simulink model "ACC_adptv_MPC_augment_constr_accel_inpt_ateteemp"  (R2024a)
settings: Solver=FixedStepAuto  StartTime=0  StopTime=100  FixedStep=.05  RelTol=1e-3
undefined symbols (not defined in the file or in its folder): act_t_delay, aero_const, ctrl_batch, Defined, delta_U_max, delta_U_min, driver_set_spd, Ego, Lane, m, matlabshared, N, Qbar, Rbar, simStepSize, state_batch, U_max, U_min, User, Y_max, Y_min
libraries: roadrunnerscenario x4, drivingscenarioandsensors x1, autolibshared x1
settings Model: PacingRate=10  Creator=darkh  LastModifiedBy=darkh
settings DataIOCC: ReturnWorkspaceOutputsName=sltest_internal_rrSimulationOutputVariable
settings DebuggingCC: AlgebraicLoopMsg=none
settings RTWCC: GPUComputeCapability=3.5
settings ConfigComp: CovSaveName=sltest_covdata  CovMetricSettings=dcmwe  CovEnableCumulative=off  CovSaveSingleToWorkspaceVar=on  CovSaveOutputData=off

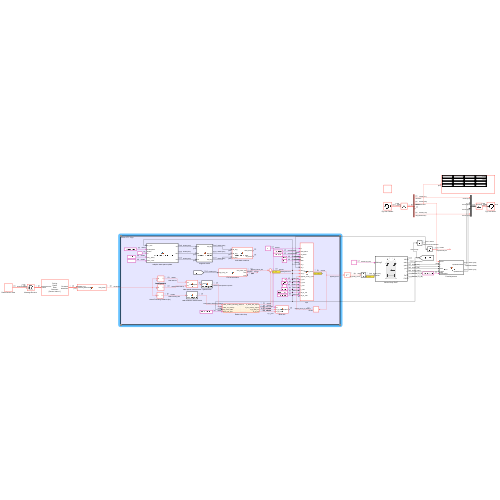
[thumbnail: Simulink's stored preview of the top-level diagram]
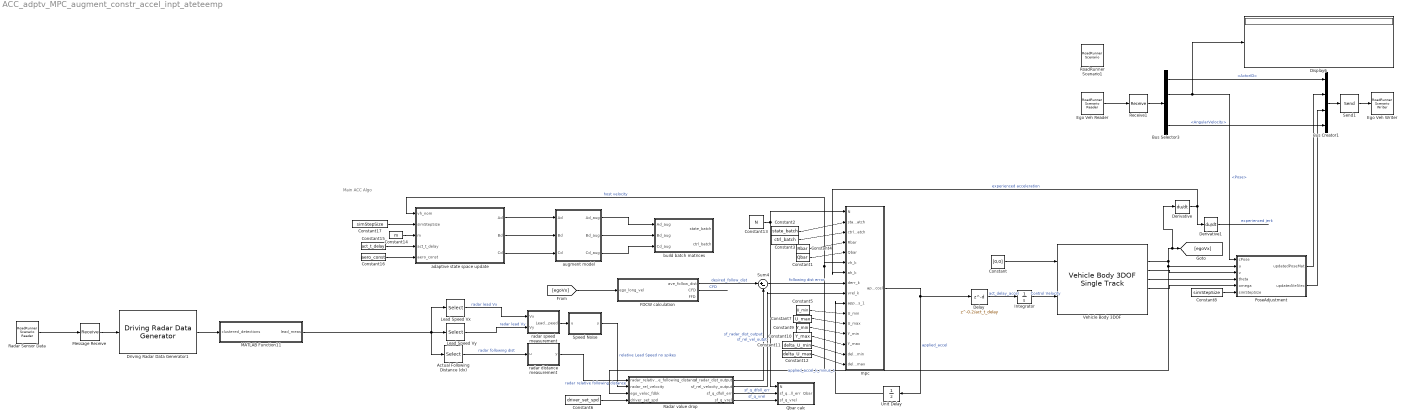
== system ACC_adptv_MPC_augment_constr_accel_inpt_ateteemp ==
  note: Main ACC Algo
  Actual Following Distance (dx) : Selector  InputPortWidth=6  IndexOptions=Index vector (dialog)  Indices=[1]  OutputSizes=1
  Bus Creator1 : BusCreator  Inputs=4  OutDataTypeStr=Bus: BusActorRuntime  NonVirtualBus=on
      settings: InheritFromInputs=off
  Bus Selector3 : BusSelector  OutputSignals=ActorID,Pose,Velocity,AngularVelocity
  Constant : Constant  Value=[0,0]
  Constant1 : Constant  Value=Qbar
  Constant10 : Constant  Value=Y_max
  Constant11 : Constant  Value=delta_U_min
  Constant12 : Constant  Value=delta_U_max
  Constant13 : Constant  Value=N
  Constant14 : Constant  Value=m
  Constant15 : Constant  Value=act_t_delay
  Constant16 : Constant  Value=aero_const
  Constant17 : Constant  Value=simStepSize
  Constant2 : Constant  Value=state_batch
  Constant3 : Constant  Value=ctrl_batch
  Constant4 : Constant  Value=Rbar
  Constant5 : Constant  Value=U_min
  Constant6 : Constant  Value=driver_set_spd
  Constant7 : Constant  Value=U_max
  Constant8 : Constant  Value=simStepSize
  Constant9 : Constant  Value=Y_min
  Delay : Delay  DelayLength=0.2/act_t_delay
  Derivative : Derivative
  Derivative1 : Derivative
  Display6 : Display
  Driving Radar Data Generator1 : drivingscenarioandsensors/Driving Radar Data Generator  SensorIndex=1  UpdateRate=20  MountingLocation=[ 3.4, 0, 0.2 ]  MountingAngles=[0 0 0]  HasElevation=off  HasRangeRate=on  HasNoise=on  HasFalseAlarms=on  HasOcclusion=on  MaxNumReportsSource=Property  MaxNumReports=50  TargetReportFormat=Clustered detections  DetectionCoordinates=Body  TrackCoordinates=Body  BusNameSource=Auto  BusName=BusDrivingRadarDataGenerator  AzimuthResolution=4  ElevationResolution=5  RangeResolution=2.5  RangeRateResolution=0.5  AzimuthBiasFraction=0.1  ElevationBiasFraction=0.1  RangeBiasFraction=0.05  RangeRateBiasFraction=0.05  FieldOfView=[ 20, 5 ]  RangeLimits=[ 0, 150 ]  RangeRateLimits=[ -100, 100 ]  DetectionProbability=0.9  FalseAlarmRate=1e-06  ReferenceRange=100  ReferenceRCS=0  CenterFrequency=77e9  FilterInitializationFcn=initcvekf  ConfirmationThreshold=[2 3]  DeletionThreshold=[5 5]  InitialSeedSource=Repeatable  InitialSeed=0  UsedSeed=matlabshared.tracking.internal.SimulinkUtilities.seedManager(gcb)  ProfilesSource=From Scenario Reader block  ProfilesParameters=driving.internal.ActorProfilesRadarParameters  ProfilesExpression=struct('ClassID',0,'Length',4.7,'Width',1.8,'Height',1.4,'OriginOffset',[-1.35 0 0],'RCSPattern',[10 10;10 10],'RCSAzimuthAngles',[-180 180],'RCSElevationAngles',[-90 90])
  Ego Veh Reader : roadrunnerscenario/RoadRunner Scenario Reader  TopicCategory=Actor  ActorCategory=All Types  ActionType=Path Following  EventType=User-Defined  TopicType=Actor Pose  VehicleType=Vehicle Specifications  UserDefinedAction=Action1  UserDefinedEvent=Event1  Filter=Self  SensorTopic=Target Poses  LaneBoundaryOutputTopic=Ego-Lane  SensorID=1  SampleTime=simStepSize
  Ego Veh Writer : roadrunnerscenario/RoadRunner Scenario Writer  TopicCategory=Actor  ActorCategory=All Types  EventType=Action Complete  UserDefinedEvent=Event1  VehicleType=Vehicle Pose  TopicType=Actor Pose
  FDCW calculation : MATLAB Function  TreatAsAtomicUnit=on
  Integrator : Integrator
  Lead Speed Vx : Selector  InputPortWidth=6  IndexOptions=Index vector (dialog)  Indices=4  OutputSizes=1
  Lead Speed Vy : Selector  InputPortWidth=6  IndexOptions=Index vector (dialog)  Indices=5  OutputSizes=1
  MATLAB Function11 : MATLAB Function  TreatAsAtomicUnit=on
  Message Receive : Receive  InputPortMessageModes=m  UseInternalQueue=off
  PoseAdjustment : MATLAB Function  TreatAsAtomicUnit=on
  Qbar calc : MATLAB Function  TreatAsAtomicUnit=on  SystemSampleTime=simStepSize
  Radar Sensor Data : roadrunnerscenario/RoadRunner Scenario Reader  TopicCategory=Sensor  ActorCategory=All Types  ActionType=Path Following  EventType=User-Defined  TopicType=Actor Specifications  VehicleType=Vehicle Specifications  UserDefinedAction=Action1  UserDefinedEvent=Event1  Filter=Self  SensorTopic=Target Poses  LaneBoundaryOutputTopic=Ego-Lane  SensorID=1  SampleTime=simStepSize
  Radar value drop : Stateflow chart  TreatAsAtomicUnit=on
  Receive1 : Receive  InputPortMessageModes=m  UseInternalQueue=off  QueueOverwriting=on  QueueLength=1  QueueType=LIFO
  RoadRunner Scenario1 : roadrunnerscenario/RoadRunner Scenario  UserDefinedActions={}  UserDefinedEvents={}
  Send1 : Send  OutputPortMessageModes=m
  Speed Noise : MATLAB Function  TreatAsAtomicUnit=on
  Sum4 : Sum  Inputs=|+-
  Unit Delay : UnitDelay  SampleTime=-1  HasFrameUpgradeWarning=on
  "Vehicle Body 3DOF " : autolibshared/Vehicle Body 3DOF Single Track  trackMode=Dual  inputMode=External longitudinal velocity  frontSteerMode=on  rearSteerMode=off  windMode=off  muMode=off  extFMode=off  extMMode=off  htchFMode=off  htchMMode=off  extXo=off  extpsio=off  extxdoto=off  extro=off  extYo=off  extTamb=off  extydoto=off  aMode=2  NF=2  NR=2  m=m  a=1.5569  b=1.5371  h=0.18903  dh=1  hh=0.2  X_o=0  xdot_o=0  CalphaMode=off  sigmaMode=on  d=0  hl=0  w=[1.4,1.4]  Cy_f=40000  Cy_r=40000  sigma_f=.1  sigma_r=.1  alpha_f_brk=[-.1 .1]  Cy_f_data=[-9e3 9e3]  alpha_r_brk=[-.1 .1]  Cy_r_data=[-9e3 9e3]  Y_o=0  ydot_o=0  Izz=2066  psi_o=0  r_o=0  Af=2.73  Cd=.30356  Cl=.1  Cpm=.1  beta_w=[0 0.01:0.01:0.3]  Cs=[0 0.01:0.01:0.3]  Cym=[0 1e-6:0.01:0.3]  Pabs=101325  Tair=273  g=9.81  mu=1  xdot_tol=.01  Fznom=5000  Fxtire_sat=7e4  Fytire_sat=7e4  longOff=0  latOff=0  vertOff=0  wrapAng=off
  adaptive state space update : MATLAB Function  TreatAsAtomicUnit=on
  augment model : MATLAB Function  TreatAsAtomicUnit=on
  build batch matrices : MATLAB Function  TreatAsAtomicUnit=on  SystemSampleTime=simStepSize
  mpc : MATLAB Function  TreatAsAtomicUnit=on  SystemSampleTime=simStepSize
  radar distance measurement : MATLAB Function  TreatAsAtomicUnit=on
  radar speed measurement : MATLAB Function  TreatAsAtomicUnit=on
  wires:
  Bus Selector3/4 -> Bus Creator1/4  "<AngularVelocity>"
  Bus Creator1/1 -> Send1/1
  Bus Selector3/1 -> Bus Creator1/1  "<ActorID>"
  Receive1/1 -> Bus Selector3/1
  Send1/1 -> Ego Veh Writer/1
  Ego Veh Reader/1 -> Receive1/1
  Bus Selector3/2 -> Display6/1, PoseAdjustment/1(cPose)  "<Pose>"
  PoseAdjustment/1(updatedPoseMat) -> Bus Creator1/2
  "Vehicle Body 3DOF "/2 -> PoseAdjustment/2(u), Radar value drop/3(ego_veloc_fdbk), adaptive state space update/1(vh_nom), mpc/6(vh_k), Derivative/1, [egoVx]  "host velocity"
  Radar Sensor Data/1 -> Message Receive/1
  Message Receive/1 -> Driving Radar Data Generator1/1
  Driving Radar Data Generator1/1 -> MATLAB Function11/1(clustered_detections)
  PoseAdjustment/2(updatedVelVec) -> Bus Creator1/3
  Integrator/1 -> "Vehicle Body 3DOF "/2  "Control Velocity"
  Constant/1 -> "Vehicle Body 3DOF "/1
  Sum4/1 -> mpc/8(derr_k)  "following dist error"
  Speed Noise/1(y) -> Radar value drop/2(radar_rel_velocity)  "relative Lead Speed no spikes"
  Lead Speed Vx/1 -> radar speed measurement/1(Vx)  "radar lead Vx"
  [egoVx] -> FDCW calculation/1(ego_long_vel)
  FDCW calculation/1(ave_follow_dist) -> Sum4/1  "desired_follow_dist"
  MATLAB Function11/1(lead_meas) -> Actual Following Distance (dx)/1, Lead Speed Vx/1, Lead Speed Vy/1
  radar distance measurement/1(y) -> Radar value drop/1(radar_relative_following_distance)  "radar relative following distance"
  Lead Speed Vy/1 -> radar speed measurement/2(Vy)  "radar lead Vy"
  radar speed measurement/1(LeadSpeed) -> Speed Noise/1(u)
  FDCW calculation/2(CFD) -> ?  "CFD"
  Actual Following Distance (dx)/1 -> radar distance measurement/1(u)  "radar following dist"
  Derivative/1 -> mpc/7(ah_k), Derivative1/1  "experienced acceleration"
  Derivative1/1 -> ?  "experienced jerk"
  Constant4/1 -> mpc/4(Rbar)
  Radar value drop/1(sf_radar_dist_output) -> Sum4/2  "sf_radar_dist_output"
  Constant6/1 -> Radar value drop/4(driver_set_spd)
  Radar value drop/2(sf_rel_velocity_output) -> mpc/9(vrel_k)  "sf_rel_vel_outpt"
  Radar value drop/3(sf_q_dfoll_err) -> Qbar calc/2(sf_q_dfoll_err)  "sf_q_dfoll_err"
  Radar value drop/4(sf_q_vrel) -> Qbar calc/3(sf_q_vrel)  "sf_q_vrel"
  Unit Delay/1 -> mpc/10(applied_accel_k_minus_1)  "applied_accel_k_minus_1"
  Constant5/1 -> mpc/11(U_min)
  Constant7/1 -> mpc/12(U_max)
  Constant8/1 -> PoseAdjustment/6(simStepSize)
  Constant9/1 -> mpc/13(Y_min)
  Constant10/1 -> mpc/14(Y_max)
  Constant11/1 -> mpc/15(del_U_min)
  Constant12/1 -> mpc/16(del_U_max)
  "Vehicle Body 3DOF "/4 -> PoseAdjustment/4(theta)
  Constant1/1 -> mpc/5(Qbar)
  "Vehicle Body 3DOF "/5 -> PoseAdjustment/5(omega)
  "Vehicle Body 3DOF "/3 -> PoseAdjustment/3(v)
  mpc/1(applied_accel) -> Unit Delay/1, Delay/1  "applied_accel"
  Constant14/1 -> adaptive state space update/3(m)
  Constant15/1 -> adaptive state space update/4(act_t_delay)
  Constant16/1 -> adaptive state space update/5(aero_const)
  Constant17/1 -> adaptive state space update/2(simStepSize)
  augment model/3(Cd_aug) -> build batch matrices/3(Cd_aug)
  augment model/2(Bd_aug) -> build batch matrices/2(Bd_aug)
  augment model/1(Ad_aug) -> build batch matrices/1(Ad_aug)
  Constant13/1 -> mpc/1(N), Qbar calc/1(N)
  adaptive state space update/1(Ad) -> augment model/1(Ad)
  adaptive state space update/2(Bd) -> augment model/2(Bd)
  adaptive state space update/3(Cd) -> augment model/3(Cd)
  Constant2/1 -> mpc/2(state_batch)
  Constant3/1 -> mpc/3(ctrl_batch)
  Delay/1 -> Integrator/1  "act_delay_accel"

== matlab function ACC_adptv_MPC_augment_constr_accel_inpt_ateteemp/build batch matrices ==
  data: state_batch output; Ad_aug input; Bd_aug input; Cd_aug input; ctrl_batch output
function [state_batch,ctrl_batch] = batch_matrix_build(Ad_aug,Bd_aug,Cd_aug)
[ny1,ny2] = size(Cd_aug);
[~,nu] = size(Bd_aug);

N=20;

% Building batch matrices for MPC prediction of output states
% batch matrix for state vector
state_batch = zeros(N*ny1, ny2);
for i = 1:N
    state_batch((i-1)*ny1+1 : i*ny1, :) = Cd_aug*(Ad_aug^i);
end

% Batch matrix for control vector
ctrl_batch = zeros(N*ny1, N*nu); % pre-allocate, fixed size

Apow = eye(size(Ad_aug)); % A^0
for i = 1:N
    % first column block for row i
    ctrl_batch((i-1)*ny1+(1:ny1), 1:nu) = Cd_aug*Apow*Bd_aug;
    % copy to the right for j = 2…i
    col = nu; % offset for next column
    Apow_j = Apow;
    for j = 2:i
        Apow_j = Apow_j / Ad_aug; % A^(i-j) (cheaper than repeated power)
        ctrl_batch((i-1)*ny1+(1:ny1), (j-1)*nu+(1:nu)) = Cd_aug*Apow_j*Bd_aug;
        col = col + nu;
    end
    Apow = Apow*Ad_aug; % advance A^i
end

== matlab function ACC_adptv_MPC_augment_constr_accel_inpt_ateteemp/PoseAdjustment ==
  data: cPose input; u input; updatedPoseMat output; v input; theta input; omega input; updatedVelVec output; simStepSize input
function [updatedPoseMat, updatedVelVec] = RRPoseAdjustment(cPose, u, v, theta, omega, simStepSize)
    thetad = theta + omega*simStepSize;
    xd = (u*cos(theta) - v*sin(theta))*simStepSize;
    yd = (u*sin(theta) + v*cos(theta))*simStepSize;
    pose_mat = [cos(-thetad) -sin(-thetad) 0 (yd+cPose(1,4)); sin(-thetad) cos(-thetad) 0 (xd+cPose(2,4)); 0 0 1 0; 0 0 0 1];
    updatedPoseMat = pose_mat;
    updatedVelVec = [u*sin(theta) + v*cos(theta), u*cos(theta) - v*sin(theta), 0];
    return;
end

== matlab function ACC_adptv_MPC_augment_constr_accel_inpt_ateteemp/radar distance measurement ==
  data: u input; y output
function y = removeSpikes(u)

    persistent buffer;
    persistent bufferIndex;
    threshold = 2;
    % windowSize = 15;
    windowSize = 5;
    
    if isempty(buffer)
        buffer = zeros(1, windowSize);
        bufferIndex = 1;
    end
    
    % Update buffer with new value
    buffer(bufferIndex) = u;
    bufferIndex = mod(bufferIndex, windowSize) + 1;
    
    % Calculate the median of the buffer
    medVal = median(buffer);
    
    % Detect and remove spikes
    if abs(u - medVal) > threshold
        y = medVal; % Replace spike with the median value
    else
        y = u; % Keep the original value if it's not a spike
    end
end

== matlab function ACC_adptv_MPC_augment_constr_accel_inpt_ateteemp/radar speed measurement ==
  data: Vx input; LeadSpeed output; Vy input
function LeadSpeed = fcn(Vx, Vy)

if Vx == 0 && Vy == 0 
    Vx = 0.01;
    Vy = 0.01;
elseif Vy == 0
    Vy = 0.01;
elseif Vx == 0
    Vx = 0.01;
end

if Vx <= 0
    LeadSpeed = -sqrt(Vx^2 + Vy^2);
else
    LeadSpeed = sqrt(Vx^2 + Vy^2);
end

== matlab function ACC_adptv_MPC_augment_constr_accel_inpt_ateteemp/Speed Noise ==
  settings: updateMethod=DISCRETE
  data: u input; y output
function y = removeSpikes(u)
    % removeSpikes - Removes spikes from a scalar signal based on a threshold
    %
    % Inputs:
    %    u - The input signal (scalar)
    %    threshold - The threshold value to detect spikes
    %    windowSize - The size of the window for calculating the median
    %
    % Outputs:
    %    y - The filtered signal with spikes removed

    % Declare persistent variables to store past values
    persistent buffer;
    persistent bufferIndex;
    threshold = 2;
    % windowSize = 15;
    windowSize = 5;

    
    if isempty(buffer)
        buffer = zeros(1, windowSize);
        bufferIndex = 1;
    end
    
    % Update buffer with new value
    buffer(bufferIndex) = u;
    bufferIndex = mod(bufferIndex, windowSize) + 1;
    
    % Calculate the median of the buffer
    medVal = median(buffer);
    
    % Detect and remove spikes
    if abs(u - medVal) > threshold
        y = medVal; % Replace spike with the median value
    else
        y = u; % Keep the original value if it's not a spike
    end
end

== matlab function ACC_adptv_MPC_augment_constr_accel_inpt_ateteemp/MATLAB Function11 ==
  data: clustered_detections input Bus: BusRadar; lead_meas output double
function lead_meas = fcn(clustered_detections)

lead_det = clustered_detections.Detections(1);
lead_meas = lead_det.Measurement;

% relative_dist = sqrt(lead_det.Measurement(1)^2 + lead_det.Measurement(2)^2); % rel_dist = sqrt(x^2+y^2)
% relative_speed = sqrt(lead_det.Measurement(4)^2 + lead_det.Measurement(5)^2);
end

== matlab function ACC_adptv_MPC_augment_constr_accel_inpt_ateteemp/FDCW calculation ==
  settings: updateMethod=DISCRETE
  data: ego_long_vel input; ave_follow_dist output; CFD output; FFD output
% Function to determine the closest (CFD) and furthest follow distance (FFD) for the
% ego vehicle relative to the lead vehicle given the ego vehicle's current
% velocity

% This function outputs the middle distance value between the CFD and FFD
% and those values respectively as well

function [ave_follow_dist, CFD, FFD] = fcn(ego_long_vel)
    persistent dist_history window_size smoothing_weights
    
    % Initialize (first call only)
    if isempty(dist_history)
        window_size = 5;  % Number of past samples
        dist_history = zeros(1, window_size);
        
        % Define and normalize weights (e.g., linear decay)
        smoothing_weights = linspace(1, 0.5, window_size);  % Weights from 1.0 to 0.5
        smoothing_weights = smoothing_weights / sum(smoothing_weights);  % Normalize
    end
    ego_long_vel_mph = ego_long_vel*2.23694;
    
    if ego_long_vel_mph > 0 && ego_long_vel_mph < 20
        CFD = 2.8*ego_long_vel_mph^0.45+8;
        FFD = 100-0.2*(20-ego_long_vel_mph)^2;
    elseif ego_long_vel_mph <= 0
        CFD = 8;
        FFD = 100-0.2*(20)^2;
    else
        CFD = 2.8*ego_long_vel_mph^0.45+8;
        FFD = 100;
    end
    AveFollowDist_Gain = 3;


    % --- Update history buffer ---
    dist_history = [ ((AveFollowDist_Gain-1)*CFD + FFD)/AveFollowDist_Gain , dist_history(1:end-1)];  % FIFO

    % --- Smoothed average (weighted, normalized) ---
    smoothed_ave_dist = sum(dist_history .* smoothing_weights);
    
    % --- Clamp to CFD/FFD bounds ---
    ave_follow_dist = min(max(smoothed_ave_dist, CFD), FFD);
end

== matlab function ACC_adptv_MPC_augment_constr_accel_inpt_ateteemp/adaptive state space update ==
  data: vh_nom input; simStepSize input; Ad output; m input; act_t_delay input; aero_const input; Bd output; Cd output
function [Ad,Bd,Cd] = adaptive_state_space_model(vh_nom, simStepSize, m, act_t_delay, aero_const)
% multiplying A matrix term with current vehicle velocity vh_nom to update
% state space model for adaptive MPC
Ac = [0,1,0,0; -aero_const*vh_nom/(m*act_t_delay), -1/act_t_delay, 0,0;0,0,0,-1;0,-1,0,0]; % with drag term
% Ac = [0,1,0,0; 0, -1/act_t_delay, 0,0;0,0,0,-1;0,-1,0,0]; % without the velocity dependent drag term
Bc = [0;1/act_t_delay;0;0];

% Using Euler discretization to obtain the discrete time matrices from the continuous time system
Ad = eye(4) + Ac.*simStepSize;
Bd = Bc.*simStepSize;
Cd = eye(4);

== matlab function ACC_adptv_MPC_augment_constr_accel_inpt_ateteemp/mpc ==
  data: N input; state_batch input; ctrl_batch input; Rbar input; Qbar input; applied_accel output; vh_k input; ah_k input; derr_k input; vrel_k input; applied_accel_k_minus_1 input; U_min input; U_max input; Y_min input; Y_max input; del_U_min input; del_U_max input
function applied_accel  = mpc(N, state_batch, ctrl_batch, Rbar, Qbar, vh_k, ah_k, derr_k, vrel_k, applied_accel_k_minus_1, U_min, U_max, Y_min, Y_max, del_U_min, del_U_max)
% Defining MPC and system variables
num_ctrl = 1;

state_vec_curr = [vh_k, ah_k, derr_k, vrel_k, applied_accel_k_minus_1]';

H = 2*(ctrl_batch' * Qbar * ctrl_batch + Rbar); % symmetric Hessian
% tiny regulariser to ensure positive-definite
H = (H+H.')/2 + 1e-8*eye(size(H));

f = 2*(ctrl_batch' * Qbar * state_batch * state_vec_curr);

persistent del_Uopt_k_minus_1 % defining persistent variable to keep track of computed optimal control signal from previous iteration
if isempty(del_Uopt_k_minus_1)
    % del_Uopt_k_minus_1 = [0,0,0,0,0,0,0,0,0,0]'; % for N = 10
    del_Uopt_k_minus_1 = [0,0,0,0,0,0,0,0,0,0,0,0,0,0,0,0,0,0,0,0]'; % for N = 20
end

%% Defining the control input limits on delta_u based on limits on u

% Determining U(k-1) from the previous control signal u(k-1) and the previous full predicted control signal delta_Uopt(k-1)
Ubar_k_minus_1 = zeros(N*num_ctrl, 1); % Initializing
Ubar_k_minus_1(1:num_ctrl,:) = applied_accel_k_minus_1; % Populating the first control vector in Uopt(k-1) as u(k-1) = [accel_app(k-1)]'

for i = 1:N-1
    Ubar_k_minus_1(i*num_ctrl+1 : (i+1)*num_ctrl, :) = Ubar_k_minus_1((i-1)*num_ctrl+1 : i*num_ctrl, :) + del_Uopt_k_minus_1(i*num_ctrl+1 : (i+1)*num_ctrl, :); % performing u(k) = u(k-1) + delta_u(k-1) for all elements to populate Uopt(k-1)
end

% Constraints on input: applied acceleration
A_qp_inpts = [eye(num_ctrl*N); -eye(num_ctrl*N)]; % both lower and upper acceleration bounds for inputs
b_qp_inpts = [U_max - Ubar_k_minus_1; -U_min + Ubar_k_minus_1];

% A_qp_inpts = [-eye(num_ctrl*N)];  % only lower bounds for inputs
% b_qp_inpts = [-U_min + Ubar_k_minus_1];

% Constraints on feeoutputs vh, ah, dfoll_err, vrel
A_qp_otpts = [ctrl_batch;-ctrl_batch]; % Both upper and lower bounds for outputs
b_qp_otpts = [Y_max - state_batch*state_vec_curr; -Y_min + state_batch*state_vec_curr];

% A_qp_otpts = [-ctrl_batch]; % only lower bounds for outputs
% b_qp_otpts = [-Y_min + state_batch*state_vec_curr];

A_qp = [A_qp_inpts; A_qp_otpts];
b_qp = [b_qp_inpts; b_qp_otpts]; 

% code where quadprog is used to solve the optimization problem
options = optimoptions('quadprog','Algorithm','active-set'); % options for quadprog
delta_Uopt = quadprog(H,f,A_qp,b_qp,[],[],del_U_min,del_U_max,del_Uopt_k_minus_1,options); % includes constraints on delta_u here

% code where mpcInteriorPointSolver is used to solve the optimization problem
% options = mpcInteriorPointOptions; % options for mpcInteriorPointSolver
% delta_Uopt = mpcInteriorPointSolver(H,f,A_qp,b_qp,zeros(0,N*num_ctrl),zeros(0,1),del_Uopt_k_minus_1,options); % does not include constraints on delta_u here

del_Uopt_k_minus_1 = delta_Uopt; % saving computed control signal for optimal delta U (over prediction horizon) for use in next iteration; becomes next delta_Uopt(k-1)

delta_u_apply = delta_Uopt(1:num_ctrl,:); % nu = number of inputs; receding horizon so only selecting the first control vector in collection to apply to plant

applied_accel = applied_accel_k_minus_1 + delta_u_apply; % Adding to previous control input since state space model is augmented to determine delta_u

== stateflow chart ACC_adptv_MPC_augment_constr_accel_inpt_ateteemp/Radar value drop ==
  state Radar_State_Lead_Veh_Present_and_Detected
    sf_radar_dist_output = radar_relative_following_distance;
    sf_rel_velocity_output = radar_rel_velocity;
    sf_q_dfoll_err = 100;
    sf_q_vrel = 100;
  state Output_Spoof_To_Keep_Moving
    sf_radar_dist_output = 100;
    set_spd_err = driver_set_spd - ego_veloc_fdbk;
    sf_rel_velocity_output = set_spd_err;
    sf_q_dfoll_err = 0;
    sf_q_vrel = 40;
  (default) -> Radar_State_Lead_Veh_Present_and_Detected
  Radar_State_Lead_Veh_Present_and_Detected -> Output_Spoof_To_Keep_Moving : [radar_relative_following_distance == 0 && radar_rel_velocity < 0.9]
  Output_Spoof_To_Keep_Moving -> Radar_State_Lead_Veh_Present_and_Detected : [radar_relative_following_distance > 0]
  data: radar_relative_following_distance input; sf_radar_dist_output output; radar_rel_velocity input; ego_veloc_fdbk input; sf_rel_velocity_output output; driver_set_spd input; set_spd_err local; sf_q_dfoll_err output; sf_q_vrel output

== matlab function ACC_adptv_MPC_augment_constr_accel_inpt_ateteemp/Qbar calc ==
  data: N input; sf_q_dfoll_err input; Qbar output; sf_q_vrel input
function Qbar = fcn(N, sf_q_dfoll_err, sf_q_vrel) 
    N = 5;
    q_vh = 0;
    q_ah = 20;
    % q_dfoll = 1000; % Set from stateflow
    % q_vrel = 100;
    
    Q = diag([q_vh, q_ah, sf_q_dfoll_err, sf_q_vrel]);
    Qbar = kron(eye(N),Q);

== matlab function ACC_adptv_MPC_augment_constr_accel_inpt_ateteemp/augment model ==
  data: Ad input; Ad_aug output; Bd input; Cd input; Bd_aug output; Cd_aug output
function [Ad_aug,Bd_aug,Cd_aug] = augment_ss_model(Ad,Bd,Cd)
[num_states,~] = size(Ad); % number of states in unaugmented system model
[~,num_ctrl] = size(Bd); % number of control inputs to system
[num_outpts,~] = size(Cd); % number of outputs from system

% Augmenting the State space model to have control vector delta_u and new state vec [x(k)', u(k-1)]' and output vec y(k) = x(k) 
Ad_aug = [Ad, Bd; zeros([num_ctrl num_states]), eye(num_ctrl)];
Bd_aug = [Bd; eye(num_ctrl)];
Cd_aug = [Cd, zeros([num_outpts num_ctrl])];
